simulink model "trafficstateflow"  (R2018b)
settings: Solver=FixedStepDiscrete  StartTime=0.0  StopTime=inf  RelTol=1e-3  EnableMultiTasking=on
settings Model: Creator=hp  LastModifiedBy=asmaa
settings OptimizationCC: DefaultParameterBehavior=Inlined  LifeSpan=1
settings DebuggingCC: UnderspecifiedInitializationDetection=Classic  MergeDetectMultiDrivingBlocksExec=none  SFUnexpectedBacktrackingDiag=warning  SFNoUnconditionalDefaultTransitionDiag=warning
settings ModelReferenceCC: PropagateSignalLabelsOutOfModel=off
settings SFSimCC: SimUseLocalCustomCode=off  MATLABDynamicMemAlloc=off
settings RTWCC: SystemTargetFile=ert.tlc  GenCodeOnly=on  TemplateMakefile=ert_default_tmf  GenerateReport=on  RTWUseLocalCustomCode=off  IncludeHyperlinkInReport=on  LaunchReport=on  GenerateTraceInfo=on  GenerateTraceReport=on  GenerateTraceReportSl=on  GenerateTraceReportSf=on  GenerateTraceReportEml=on
settings CodeAppCC: ForceParamTrailComments=on  IgnoreCustomStorageClasses=off  OperatorAnnotations=on  SimulinkDataObjDesc=on  SFDataObjDesc=on  MATLABFcnDesc=on  InsertBlockDesc=on  StateflowObjectComments=on  MATLABSourceComments=on
settings ERTTargetCC: MultiwordLength=2048  GenerateSampleERTMain=on  InlinedParameterPlacement=NonHierarchical  ERTCustomFileTemplate=example_file_process.tlc
settings ConfigComp: CovMetricSettings=dw  CovHtmlReporting=on  CovSaveCumulativeToWorkspaceVar=on  CovSaveSingleToWorkspaceVar=on  CovExternalEMLEnable=off
settings SimscapeCC: SimscapeNormalizeSystem=off

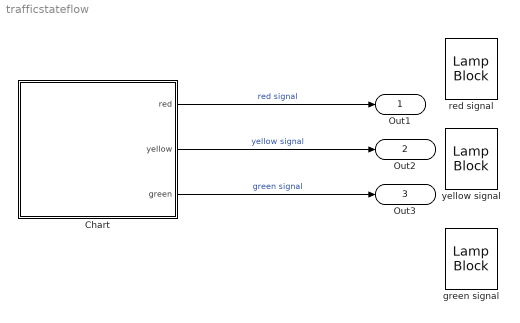
== system trafficstateflow ==
  Chart : Stateflow chart  TreatAsAtomicUnit=on
  green signal : LampBlock  WebBlockId=40
  red signal : LampBlock  WebBlockId=38
  yellow signal : LampBlock  WebBlockId=39
  Out1 : Outport
  Out2 : Outport  Port=2
  Out3 : Outport  Port=3
  wires:
  Chart/3(green) -> Out3/1  "green signal"
  Chart/2(yellow) -> Out2/1  "yellow signal"
  Chart/1(red) -> Out1/1  "red signal"

== stateflow chart trafficstateflow/Chart ==
  state Stop_
    en:
    red = uint8(0);
    yellow = uint8(0);
    green = uint8(0);
    du:
    red = uint8(1);
    yellow = uint8(0);
    green = uint8(0);
    ex:
  state Ready_
    en:
    red = uint8(0);
    yellow = uint8(0);
    green = uint8(0);
    du:
    red = uint8(0);
    yellow = uint8(1);
    green = uint8(0);
    ex:
  state Green_
    en:
    red = uint8(0);
    yellow = uint8(0);
    green = uint8(0);
    du:
    red = uint8(0);
    yellow = uint8(0);
    green = uint8(1);
    ex:
  (default) -> Stop_
  Stop_ -> Ready_ : after(3000,msec)
  Green_ -> Stop_ : after(3000,msec)
  Ready_ -> Green_ : after(3000,msec)
  data: red output uint8; yellow output uint8; green output uint8
